simulink model "fm_radio_simulink_v4"  (R2025b)
settings: Solver=FixedStepDiscrete  StartTime=0.0  StopTime=SimTime  RelTol=1e-3
undefined symbols (not defined in the file): a_de, b_de, CoefFilter1, CoefFilter2, CoefFilter3, CoefFilter4, fs_rf, rx_iq
libraries: dsphdlfiltering2 x4, dspsrcs4 x2
settings Model: DataTypeOverride=Off  SimulationMode=accelerator  Creator=kmuws  LastModifiedBy=kmuws
settings OptimizationCC: BlockReduction=off  ConditionallyExecuteInputs=off  DefaultParameterBehavior=Inlined  InheritOutputTypeSmallerThanSingle=on
settings DebuggingCC: ArtificialAlgebraicLoopMsg=error  SingleTaskRateTransMsg=error
settings HardwareCC: ProdBitPerPointer=32.0  ProdBitPerSizeT=32.0  ProdBitPerPtrDiffT=32.0  ProdLargestAtomicFloat=None  ProdIntDivRoundTo=Undefined  ProdEndianess=Unspecified  ProdWordSize=32.0  ProdHWDeviceType=ASIC/FPGA->ASIC/FPGA  TargetBitPerLong=64.0  TargetBitPerPointer=64.0  TargetBitPerSizeT=64.0  TargetBitPerPtrDiffT=64.0  TargetLongLongMode=on  TargetIntDivRoundTo=Zero  TargetEndianess=LittleEndian  TargetWordSize=64.0  TargetHWDeviceType=Custom Processor->MATLAB Host Computer  ProdEqTarget=off

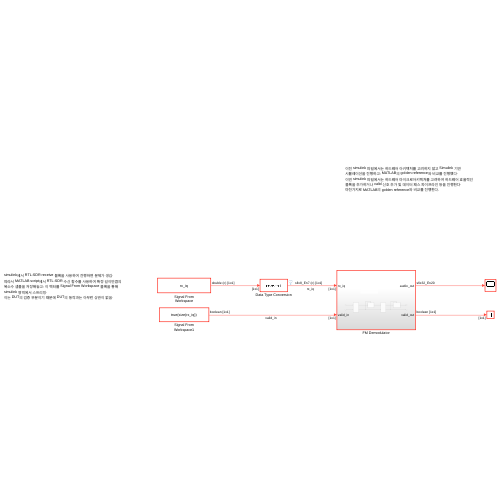
[thumbnail: Simulink's stored preview of the top-level diagram]
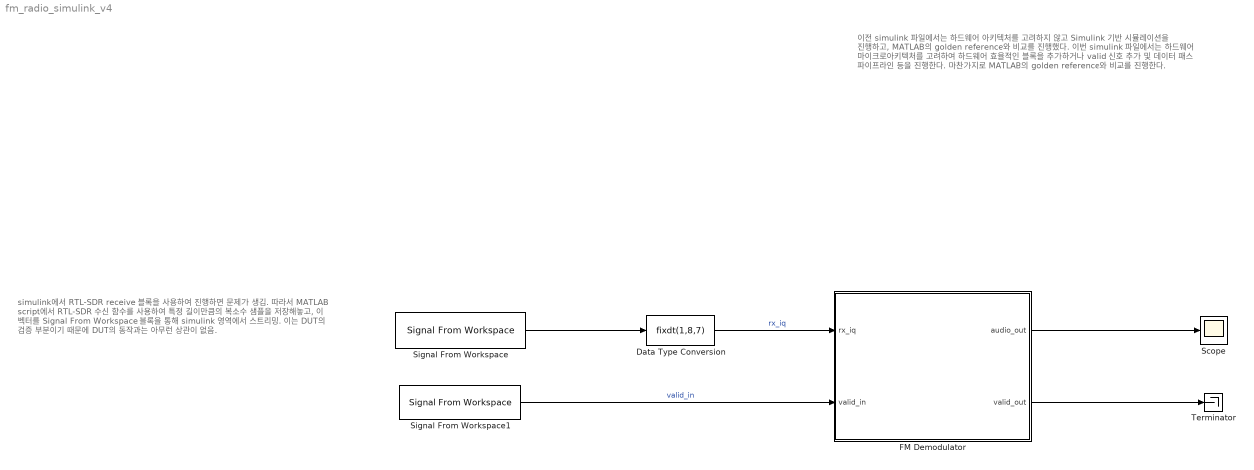
== system fm_radio_simulink_v4 ==
  note: 이전 simulink 파일에서는 하드웨어 아키텍처를 고려하지 않고 Simulink 기반
      | 시뮬레이션을 진행하고, MATLAB의 golden reference와 비교를 진행했다.
      | 이번 simulink 파일에서는 하드웨어 마이크로아키텍처를 고려하여 하드웨어 효율적인
      | 블록을 추가하거나 valid 신호 추가 및 데이터 패스 파이프라인 등을 진행한다.
      | 마찬가지로 MATLAB의 golden reference와 비교를 진행한다.
  note: simulink에서 RTL-SDR receive 블록을 사용하여 진행하면 문제가 생김.
      | 따라서 MATLAB script에서 RTL-SDR 수신 함수를 사용하여 특정 길이만큼의
      | 복소수 샘플을 저장해놓고, 이 벡터를 Signal From Workspace 블록을 통해
      | simulink 영역에서 스트리밍.
      | 이는 DUT의 검증 부분이기 때문에 DUT의 동작과는 아무런 상관이 없음.
  Data Type Conversion : DataTypeConversion  OutDataTypeStr=fixdt(1,8,7)  SaturateOnIntegerOverflow=off  RndMeth=Floor
  FM Demodulator : Subsystem
  Scope : Scope
      settings: ActiveDisplayYMinimum=-0.65770959854125977  ActiveDisplayYMaximum=0.60501718521118164
  Signal From Workspace : dspsrcs4/Signal From Workspace  X=rx_iq  Ts=1/fs_rf  nsamps=1  OutputAfterFinalValue=Setting to zero  ignoreOrWarnInputAndFrameLengths=off  OutputFrames=off
  Signal From Workspace1 : dspsrcs4/Signal From Workspace  X=true(size(rx_iq))  Ts=1/fs_rf  nsamps=1  OutputAfterFinalValue=Setting to zero  ignoreOrWarnInputAndFrameLengths=off  OutputFrames=off
  Terminator : Terminator
  wires:
  FM Demodulator/1(audio_out) -> Scope/1
  FM Demodulator/2(valid_out) -> Terminator/1
  Data Type Conversion/1 -> FM Demodulator/1(rx_iq)  "rx_iq"
  Signal From Workspace/1 -> Data Type Conversion/1
  Signal From Workspace1/1 -> FM Demodulator/2(valid_in)  "valid_in"

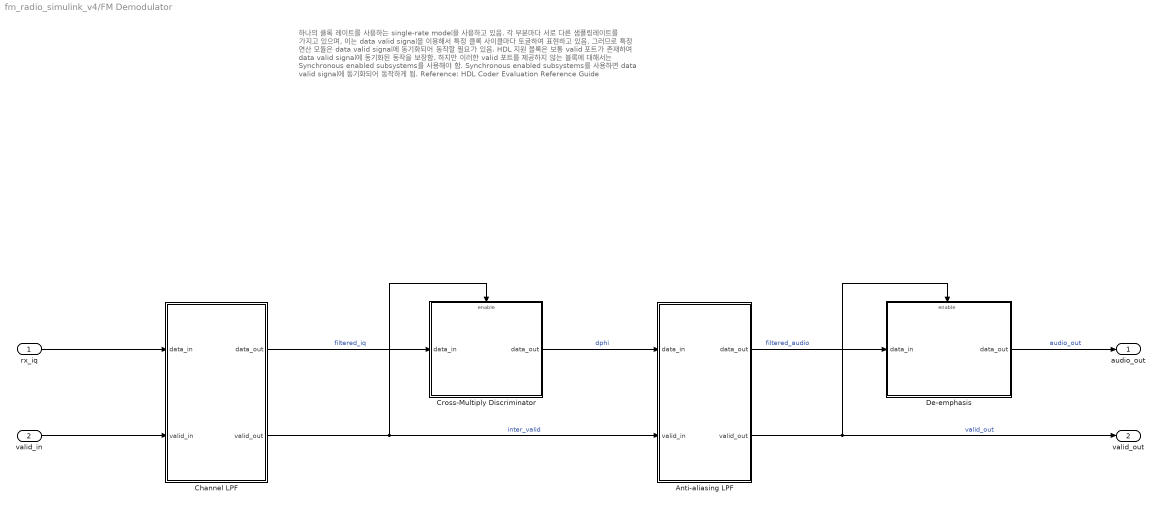
== system fm_radio_simulink_v4/FM Demodulator ==
  note: 하나의 클록 레이트를 사용하는 single-rate model을 사용하고 있음.
      | 각 부분마다 서로 다른 샘플링레이트를 가지고 있으며, 이는 data valid signal을 이용해서 특정 클록 사이클마다 토글하여 표현하고 있음.
      | 그러므로 특정 연산 모듈은 data valid signal에 동기화되어 동작할 필요가 있음.
      | HDL 지원 블록은 보통 valid 포트가 존재하여 data valid signal에 동기화된 동작을 보장함. 하지만 이러한 valid 포트를 제공하지 않는 블록에 대해서는 Synchronous enabled subsystems를 사용해야 함.
      | Synchronous enabled subsystems를 사용하면 data valid signal에 동기화되어 동작하게 됨.
      |
      | Reference: HDL Coder Evaluation Reference Guide
  rx_iq : Inport
  valid_in : Inport  Port=2
  Anti-aliasing LPF : Subsystem
  Channel LPF : Subsystem
  Cross-Multiply Discriminator : Subsystem  TreatAsAtomicUnit=on
  De-emphasis : Subsystem  TreatAsAtomicUnit=on
  audio_out : Outport
  valid_out : Outport  Port=2
  wires:
  Anti-aliasing LPF/2(valid_out) -> valid_out/1, De-emphasis/Enable  "valid_out"
  rx_iq/1 -> Channel LPF/1(data_in)
  valid_in/1 -> Channel LPF/2(valid_in)
  Channel LPF/1(data_out) -> Cross-Multiply Discriminator/1(data_in)  "filtered_iq"
  Channel LPF/2(valid_out) -> Anti-aliasing LPF/2(valid_in), Cross-Multiply Discriminator/Enable  "inter_valid"
  Anti-aliasing LPF/1(data_out) -> De-emphasis/1(data_in)  "filtered_audio"
  Cross-Multiply Discriminator/1(data_out) -> Anti-aliasing LPF/1(data_in)  "dphi"
  De-emphasis/1(data_out) -> audio_out/1  "audio_out"

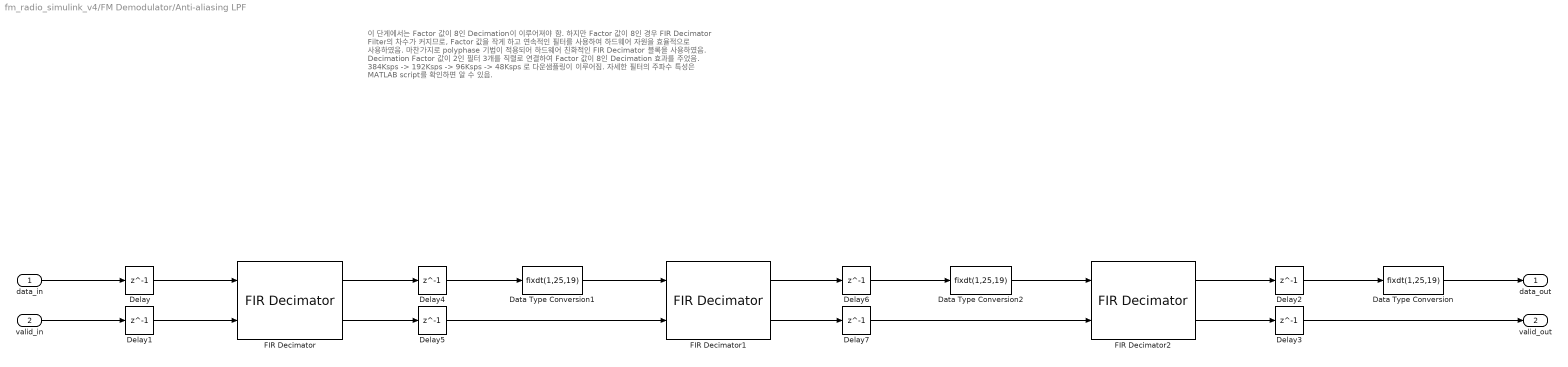
== system fm_radio_simulink_v4/FM Demodulator/Anti-aliasing LPF ==
  note: 이 단게에서는 Factor 값이 8인 Decimation이 이루어져야 함. 하지만 Factor 값이 8인 경우 FIR Decimator Filter의 차수가 커지므로, Factor 값을 작게 하고 연속적인 필터를 사용하여 하드웨어 자원을 효율적으로 사용하였음.
      | 마찬가지로 polyphase 기법이 적용되어 하드웨어 친화적인 FIR Decimator 블록을 사용하였음.
      | Decimation Factor 값이 2인 필터 3개를 직렬로 연결하여 Factor 값이 8인 Decimation 효과를 주었음. 384Ksps -> 192Ksps -> 96Ksps -> 48Ksps로 다운샘플링이 이루어짐.
      | 자세한 필터의 주파수 특성은 MATLAB script를 확인하면 알 수 있음.
  data_in : Inport
  valid_in : Inport  Port=2
  Data Type Conversion : DataTypeConversion  OutDataTypeStr=fixdt(1,25,19)  SaturateOnIntegerOverflow=off  RndMeth=Floor
  Data Type Conversion1 : DataTypeConversion  OutDataTypeStr=fixdt(1,25,19)  SaturateOnIntegerOverflow=off  RndMeth=Floor
  Data Type Conversion2 : DataTypeConversion  OutDataTypeStr=fixdt(1,25,19)  SaturateOnIntegerOverflow=off  RndMeth=Floor
  Delay{,1..7} (8 alike) : Delay  DelayLength=1  InitialCondition=0
  FIR Decimator : dsphdlfiltering2/FIR Decimator  NumeratorSource=Property  Numerator=CoefFilter2  NumeratorPrototype=[]  FilterStructure=Direct form systolic  DecimationFactor=decim2  NumCycles=1  OptimizeSymmCoeff=on  SimulateUsing=Code generation  roundingMode=Floor  overflowMode=off  CoefficientsDataTypeStr=fixdt(1,18,17)  ResetInputPort=off  HDLGlobalReset=off
  FIR Decimator1 : dsphdlfiltering2/FIR Decimator  NumeratorSource=Property  Numerator=CoefFilter3  NumeratorPrototype=[]  FilterStructure=Direct form systolic  DecimationFactor=decim3  NumCycles=1  OptimizeSymmCoeff=on  SimulateUsing=Code generation  roundingMode=Floor  overflowMode=off  CoefficientsDataTypeStr=fixdt(1,18,17)  ResetInputPort=off  HDLGlobalReset=off
  FIR Decimator2 : dsphdlfiltering2/FIR Decimator  NumeratorSource=Property  Numerator=CoefFilter4  NumeratorPrototype=[]  FilterStructure=Direct form systolic  DecimationFactor=decim4  NumCycles=1  OptimizeSymmCoeff=on  SimulateUsing=Code generation  roundingMode=Floor  overflowMode=off  CoefficientsDataTypeStr=fixdt(1,18,17)  ResetInputPort=off  HDLGlobalReset=off
  data_out : Outport
  valid_out : Outport  Port=2
  wires:
  data_in/1 -> Delay/1
  FIR Decimator2/1 -> Delay2/1
  valid_in/1 -> Delay1/1
  FIR Decimator2/2 -> Delay3/1
  Delay/1 -> FIR Decimator/1
  Delay1/1 -> FIR Decimator/2
  Delay2/1 -> Data Type Conversion/1
  Delay3/1 -> valid_out/1
  Data Type Conversion/1 -> data_out/1
  FIR Decimator/1 -> Delay4/1
  FIR Decimator/2 -> Delay5/1
  Delay4/1 -> Data Type Conversion1/1
  FIR Decimator1/2 -> Delay7/1
  FIR Decimator1/1 -> Delay6/1
  Delay6/1 -> Data Type Conversion2/1
  Delay7/1 -> FIR Decimator2/2
  Data Type Conversion1/1 -> FIR Decimator1/1
  Delay5/1 -> FIR Decimator1/2
  Data Type Conversion2/1 -> FIR Decimator2/1

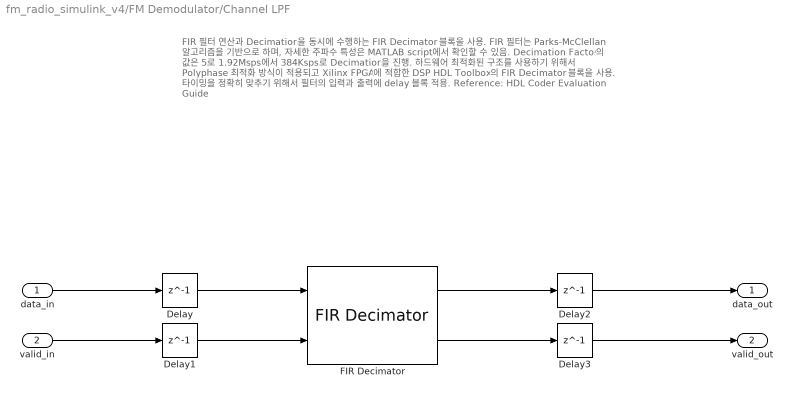
== system fm_radio_simulink_v4/FM Demodulator/Channel LPF ==
  note: FIR 필터 연산과 Decimation을 동시에 수행하는 FIR Decimator 블록을 사용.
      | FIR 필터는 Parks-McClellan 알고리즘을 기반으로 하며, 자세한 주파수 특성은 MATLAB script에서 확인할 수 있음.
      | Decimation Factor의 값은 5로 1.92Msps에서 384Ksps로 Decimation을 진행.
      | 하드웨어 최적화된 구조를 사용하기 위해서 Polyphase 최적화 방식이 적용되고 Xilinx FPGA에 적합한 DSP HDL Toolbox의 FIR Decimator 블록을 사용.
      |
      | 타이밍을 정확히 맞추기 위해서 필터의 입력과 출력에 delay 블록 적용.
      |
      | Reference: HDL Coder Evaluation Guide
  data_in : Inport
  valid_in : Inport  Port=2
  Delay{,1..3} (4 alike) : Delay  DelayLength=1  InitialCondition=0
  FIR Decimator : dsphdlfiltering2/FIR Decimator  NumeratorSource=Property  Numerator=CoefFilter1  NumeratorPrototype=[]  FilterStructure=Direct form systolic  DecimationFactor=decim1  NumCycles=1  OptimizeSymmCoeff=on  SimulateUsing=Code generation  roundingMode=Floor  overflowMode=off  CoefficientsDataTypeStr=fixdt(1,18,17)  ResetInputPort=off  HDLGlobalReset=off
  data_out : Outport
  valid_out : Outport  Port=2
  wires:
  FIR Decimator/1 -> Delay2/1
  data_in/1 -> Delay/1
  valid_in/1 -> Delay1/1
  FIR Decimator/2 -> Delay3/1
  Delay/1 -> FIR Decimator/1
  Delay1/1 -> FIR Decimator/2
  Delay3/1 -> valid_out/1
  Delay2/1 -> data_out/1

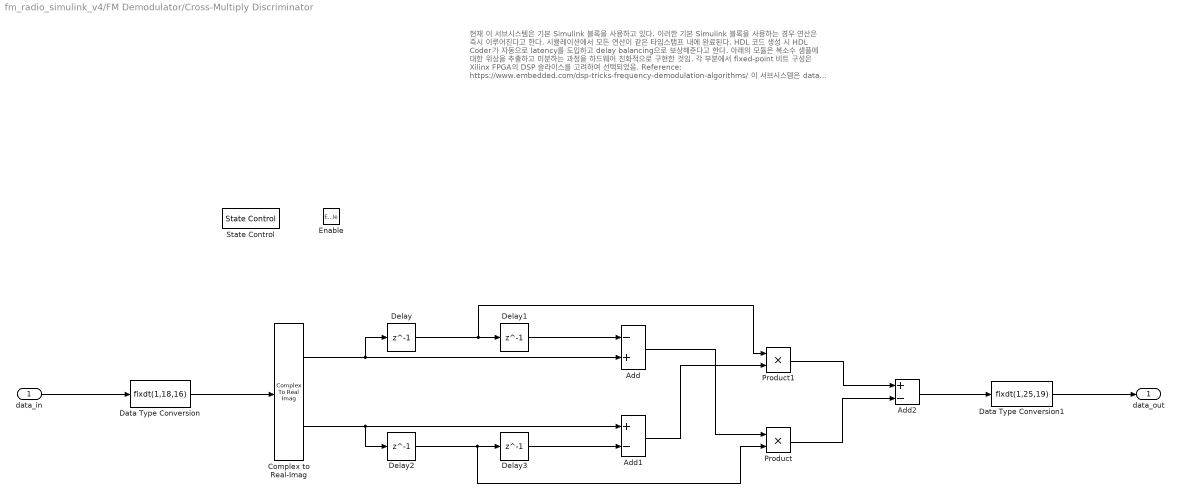
== system fm_radio_simulink_v4/FM Demodulator/Cross-Multiply Discriminator ==
  note: 현재 이 서브시스템은 기본 Simulink 블록을 사용하고 있다. 이러한 기본 Simulink 블록을 사용하는 경우 연산은 즉시 이루어진다고 한다. 시뮬레이션에서 모든 연산이 같은 타임스탬프 내에 완료된다.
      | HDL 코드 생성 시 HDL Coder가 자동으로 latency를 도입하고 delay balancing으로 보상해준다고 한다.
      |
      | 아래의 모듈은 복소수 샘플에 대한 위상을 추출하고 미분하는 과정을 하드웨어 친화적으로 구현한 것임. 각 부분에서 fixed-point 비트 구성은 Xilinx FPGA의 DSP 슬라이스를 고려하여 선택되었음.
      |
      | Reference: https://www.embedded.com/dsp-tricks-frequency-demodulation-algorithms/
      |
      | 이 서브시스템은 data valid 신호에 따라서 동작해야 함. 따라서 Synchronous Enabled Subsystems를 사용하여 유효한 데이터가 주어지는 경우에만 enabled 되도록 구현함.
      |
      | Reference: HDL Coder Evaluation Guide
  data_in : Inport
  Enable : EnablePort
  Add : Sum  Inputs=-+
  Add1 : Sum  Inputs=+-
  Add2 : Sum  Inputs=+-
  Complex to Real-Imag : ComplexToRealImag
  Data Type Conversion : DataTypeConversion  OutDataTypeStr=fixdt(1,18,16)  SaturateOnIntegerOverflow=off  RndMeth=Floor
  Data Type Conversion1 : DataTypeConversion  OutDataTypeStr=fixdt(1,25,19)  SaturateOnIntegerOverflow=off  RndMeth=Floor
  Delay{,1..3} (4 alike) : Delay  DelayLength=1  InitialCondition=0
  Product : Product
  Product1 : Product
  State Control : StateControl  StateControl=Synchronous
  data_out : Outport
  wires:
  data_in/1 -> Data Type Conversion/1
  Complex to Real-Imag/1 -> Add/2, Delay/1
  Complex to Real-Imag/2 -> Delay2/1, Add1/1
  Data Type Conversion/1 -> Complex to Real-Imag/1
  Data Type Conversion1/1 -> data_out/1
  Delay/1 -> Delay1/1, Product1/1
  Delay1/1 -> Add/1
  Delay2/1 -> Product/2, Delay3/1
  Delay3/1 -> Add1/2
  Add/1 -> Product/1
  Add1/1 -> Product1/2
  Product1/1 -> Add2/1
  Product/1 -> Add2/2
  Add2/1 -> Data Type Conversion1/1

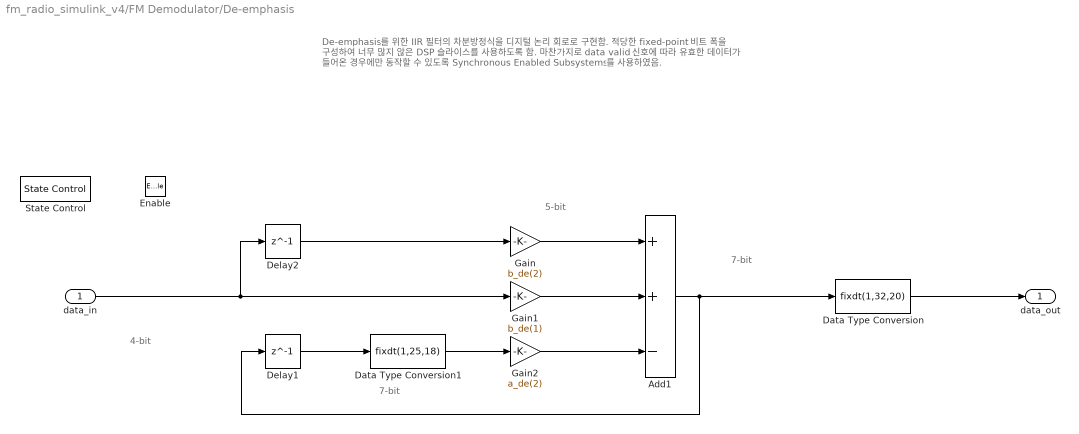
== system fm_radio_simulink_v4/FM Demodulator/De-emphasis ==
  note: De-emphasis를 위한 IIR 필터의 차분방정식을 디지털 논리 회로로 구현함.
      | 적당한 fixed-point 비트 폭을 구성하여 너무 많지 않은 DSP 슬라이스를 사용하도록 함.
      |  마찬가지로 data valid 신호에 따라 유효한 데이터가 들어온 경우에만 동작할 수 있도록 Synchronous Enabled Subsystems를 사용하였음.
  note: 7-bit
  note: 5-bit
  note: 7-bit
  note: 4-bit
  data_in : Inport
  Enable : EnablePort
  Add1 : Sum  Inputs=++-
  Data Type Conversion : DataTypeConversion  OutDataTypeStr=fixdt(1,32,20)  SaturateOnIntegerOverflow=off  RndMeth=Floor
  Data Type Conversion1 : DataTypeConversion  OutDataTypeStr=fixdt(1,25,18)  SaturateOnIntegerOverflow=off  RndMeth=Floor
  Delay1 : Delay  DelayLength=1
  Delay2 : Delay  DelayLength=1
  Gain : Gain  Gain=b_de(2)  ParamDataTypeStr=fixdt(1,25,24)
  Gain1 : Gain  Gain=b_de(1)  ParamDataTypeStr=fixdt(1,25,24)
  Gain2 : Gain  Gain=a_de(2)  ParamDataTypeStr=fixdt(1,25,24)
  State Control : StateControl  StateControl=Synchronous
  data_out : Outport
  wires:
  Delay2/1 -> Gain/1
  Gain1/1 -> Add1/2
  Add1/1 -> Data Type Conversion/1, Delay1/1
  Gain/1 -> Add1/1
  Delay1/1 -> Data Type Conversion1/1
  Gain2/1 -> Add1/3
  data_in/1 -> Gain1/1, Delay2/1
  Data Type Conversion1/1 -> Gain2/1
  Data Type Conversion/1 -> data_out/1
